simulink model "ejercicio5a"  (R2015a)
settings: Solver=ode45  StartTime=0.0  StopTime=10.0  RelTol=1e-3
settings Model: Creator=gonzalo  LastModifiedBy=gonzalo

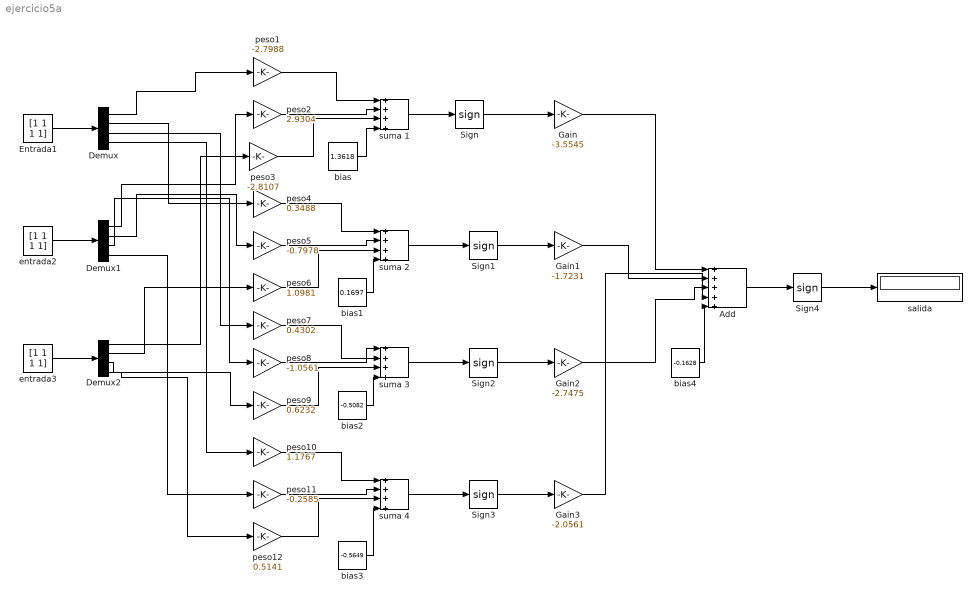
== system ejercicio5a ==
  Add : Sum  Inputs=+++++
  Demux : Demux
  Demux1 : Demux
  Demux2 : Demux
  Entrada1 : Constant  Value=[1 1 1 1]
  Gain : Gain  Gain=-3.5545
  Gain1 : Gain  Gain=-1.7231
  Gain2 : Gain  Gain=-2.7475
  Gain3 : Gain  Gain=-2.0561
  Sign{,1..4} (5 alike) : Signum
  bias : Constant  Value=1.3618
  bias1 : Constant  Value=0.1697
  bias2 : Constant  Value=-0.5082
  bias3 : Constant  Value=-0.5649
  "bias4 " : Constant  Value=-0.1628
  entrada2 : Constant  Value=[1 1 1 1]
  entrada3 : Constant  Value=[1 1 1 1]
  peso1 : Gain  Gain=-2.7988
  peso10 : Gain  Gain=1.1767
  peso11 : Gain  Gain=-0.2585
  peso12 : Gain  Gain=0.5141
  peso2 : Gain  Gain=2.9304
  peso3 : Gain  Gain=-2.8107
  peso4 : Gain  Gain=0.3488
  peso5 : Gain  Gain=-0.7978
  peso6 : Gain  Gain=1.0981
  peso7 : Gain  Gain=0.4302
  peso8 : Gain  Gain=-1.0561
  peso9 : Gain  Gain=0.6232
  salida : Display
  suma {1..4} (4 alike) : Sum  Inputs=++++
  wires:
  peso1/1 -> suma 1/1
  peso2/1 -> suma 1/2
  peso3/1 -> suma 1/3
  peso4/1 -> suma 2/1
  peso5/1 -> suma 2/2
  peso6/1 -> suma 2/3
  peso7/1 -> suma 3/1
  peso8/1 -> suma 3/2
  peso9/1 -> suma 3/3
  peso10/1 -> suma 4/1
  peso11/1 -> suma 4/2
  peso12/1 -> suma 4/3
  suma 1/1 -> Sign/1
  suma 2/1 -> Sign1/1
  suma 3/1 -> Sign2/1
  suma 4/1 -> Sign3/1
  Add/1 -> Sign4/1
  Gain/1 -> Add/1
  Gain1/1 -> Add/2
  Gain2/1 -> Add/3
  Gain3/1 -> Add/4
  Sign/1 -> Gain/1
  Sign1/1 -> Gain1/1
  Sign2/1 -> Gain2/1
  Sign3/1 -> Gain3/1
  Sign4/1 -> salida/1
  Demux/1 -> peso1/1
  Demux/2 -> peso4/1
  Demux/3 -> peso7/1
  Demux/4 -> peso10/1
  Demux1/1 -> peso2/1
  Demux1/2 -> peso5/1
  Demux1/3 -> peso8/1
  Demux1/4 -> peso11/1
  Demux2/1 -> peso3/1
  Demux2/2 -> peso6/1
  Demux2/3 -> peso9/1
  Demux2/4 -> peso12/1
  entrada3/1 -> Demux2/1
  entrada2/1 -> Demux1/1
  Entrada1/1 -> Demux/1
  bias/1 -> suma 1/4
  bias1/1 -> suma 2/4
  bias2/1 -> suma 3/4
  bias3/1 -> suma 4/4
  "bias4 "/1 -> Add/5
